simulink model "WM390_IMA_1DModel23_v2_GroupXX"  (R2021b)
settings: Solver=ode14x  StartTime=0.0  StopTime=1800  FixedStep=0.01  RelTol=1e-3
PreLoadFcn:
  | load('ACS_1DModel23_Parameters_v2.mat');
values from neighbouring files (symbols this model uses):
  AmbTemp = 25    [ACS_1DModel23_Parameters_v2.mat]
  CellContCur = 8.3    [ACS_1DModel23_Parameters_v2.mat]
  Init_SoC = 100    [ACS_1DModel23_Parameters_v2.mat]
  kI = 0.001    [ACS_1DModel23_Parameters_v2.mat]
  kP = 0.05    [ACS_1DModel23_Parameters_v2.mat]
  nP = 3    [ACS_1DModel23_Parameters_v2.mat]
  nS = 96    [ACS_1DModel23_Parameters_v2.mat]
  SoCmin = 10    [ACS_1DModel23_Parameters_v2.mat]
  ThrottleBP = [0 5 10 15 20 25 30 35 40 45 50 55 ... (21 elements, 21x1)]    [ACS_1DModel23_Parameters_v2.mat]
  TMaxMotor = 120    [ACS_1DModel23_Parameters_v2.mat]
undefined symbols (not defined in the file or in its folder): G_A, VehicleMass
libraries: nesl_utility x21, fl_lib x14, sdl_lib x8, simulink x3, autolibrcnetworksystem x1, autolibmappedmotorcommon x1, autolibshared x1
(part 1 of 2)
settings Model: PauseTimes=2  NumberOfSteps=200000  Creator=ogden.michael  LastModifiedBy=Truong Bui
settings SolverCC: AlgebraicLoopSolver=TrustRegion
settings DataIOCC: ReturnWorkspaceOutputs=off
settings OptimizationCC: EnhancedBackFolding=on  PassReuseOutputArgsThreshold=0  OptimizeBlockOrder=speed  DifferentSizesBufferReuse=on  OptimizationCustomize=off
settings DebuggingCC: AlgebraicLoopMsg=none  ParameterTunabilityLossMsg=error  SFMachineParentedDataDiag=warning  ArithmeticOperatorsInVariantConditions=warning
settings SFSimCC: SimUseLocalCustomCode=off  MATLABDynamicMemAlloc=off  CustomCodeUndefinedFunction=UseInterfaceOnly
settings RTWCC: RTWVerbose=off  RTWUseLocalCustomCode=off
settings CodeAppCC: ForceParamTrailComments=on  OperatorAnnotations=on
settings GRTTargetCC: TargetLangStandard=C89/C90 (ANSI)
settings SimscapeCC: SimscapeNormalizeSystem=off

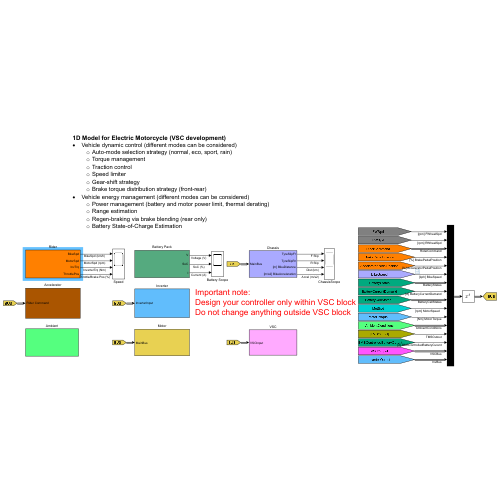
[thumbnail: Simulink's stored preview of the top-level diagram]
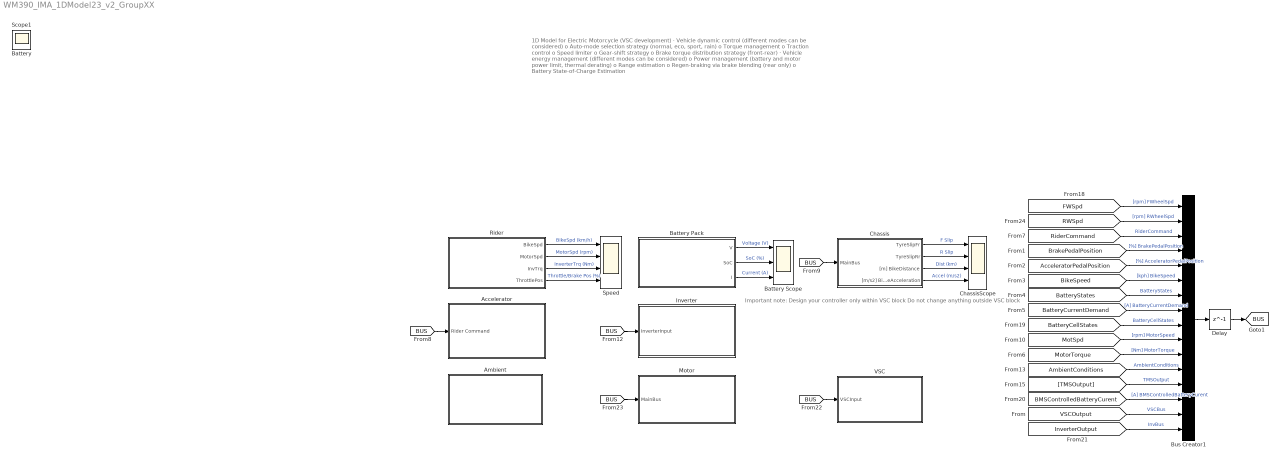
== system WM390_IMA_1DModel23_v2_GroupXX ==
  note: Important note:
      | Design your controller only within VSC block
      | Do not change anything outside VSC block
  note: 1D Model for Electric Motorcycle (VSC development)
      | · Vehicle dynamic control (different modes can be considered)
      | o Auto-mode selection strategy (normal, eco, sport, rain)
      | o Torque management
      | o Traction control
      | o Speed limiter
      | o Gear-shift strategy
      | o Brake torque distribution strategy (front-rear)
      | · Vehicle energy management (different modes can be considered)
      | o Power management (battery and motor power limit, thermal derating)
      | o Range estimation
      | o Regen-braking via brake blending (rear only)
      | o Battery State-of-Charge Estimation
  Accelerator : Subsystem
  Ambient : Subsystem
  Battery Pack : Subsystem
  Battery Scope : Scope  NumInputPorts=3
  Bus Creator1 : BusCreator  Inputs=16  OutDataTypeStr=Bus: ModelBus
      settings: InheritFromInputs=off
  Chassis : Subsystem
  ChassisScope : Scope  NumInputPorts=4
  Delay : Delay  DelayLength=1
  Inverter : Subsystem
  Motor : Subsystem
  Rider : Subsystem
  Speed : Scope  NumInputPorts=4
  VSC : Subsystem
  Battery : Scope
  Scope1 : Scope
  tag scope: BUS=global
  wires:
  [BrakePedalPosition] -> Bus Creator1/4  "[%] BrakePedalPosition"
  [AcceleratorPedalPosition] -> Bus Creator1/5  "[%] AcceleratorPedalPosition"
  [BikeSpeed] -> Bus Creator1/6  "[kph] BikeSpeed"
  [BatteryStates] -> Bus Creator1/7  "BatteryStates"
  [BatteryCurrentDemand] -> Bus Creator1/8  "[A] BatteryCurrentDemand"
  [MotorTorque] -> Bus Creator1/11  "[Nm] MotorTorque"
  [RiderCommand] -> Bus Creator1/3  "RiderCommand"
  [AmbientConditions] -> Bus Creator1/12  "AmbientConditions"
  [TMSOutput] -> Bus Creator1/13  "TMSOutput"
  [BatteryCellStates] -> Bus Creator1/9  "BatteryCellStates"
  [BMSControlledBatteryCurent] -> Bus Creator1/14  "[A] BMSControlledBatteryCurent"
  [BUS] -> Accelerator/1(Rider Command)
  [BUS] -> Inverter/1(InverterInput)
  Bus Creator1/1 -> Delay/1
  [VSCOutput] -> Bus Creator1/15  "VSCBus"
  [InverterOutput] -> Bus Creator1/16  "InvBus"
  [RWSpd] -> Bus Creator1/2  "[rpm] RWheelSpd"
  [BUS] -> Motor/1(MainBus)
  [BUS] -> VSC/1(VSCInput)
  [MotSpd] -> Bus Creator1/10  "[rpm] MotorSpeed"
  [FWSpd] -> Bus Creator1/1  "[rpm] FWheelSpd"
  Delay/1 -> [BUS]
  Chassis/3("[m] BikeDistance") -> ChassisScope/3  "Dist (km)"
  [BUS] -> Chassis/1(MainBus)
  Chassis/1(TyreSlipFr) -> ChassisScope/1  "F Slip"
  Chassis/2(TyreSlipRr) -> ChassisScope/2  "R Slip"
  Chassis/4("[m/s2] BikeAcceleration") -> ChassisScope/4  "Accel (m/s2)"
  Battery Pack/3(I) -> Battery Scope/3  "Current (A)"
  Battery Pack/2(SoC) -> Battery Scope/2  "SoC (%)"
  Battery Pack/1(V) -> Battery Scope/1  "Voltage (V)"
  Rider/3(InvTrq) -> Speed/3  "InverterTrq (Nm)"
  Rider/2(MotorSpd) -> Speed/2  "MotorSpd (rpm)"
  Rider/1(BikeSpd) -> Speed/1  "BikeSpd (km/h)"
  Rider/4(ThrottlePos) -> Speed/4  "Throttle/Brake Pos (%)"

== system WM390_IMA_1DModel23_v2_GroupXX/Accelerator ==
  Rider Command : Inport
  Accelerator Dynamics : TransferFcn  Denominator=[0.15 1]
  Accelerator Limitter : Saturate  UpperLimit=100  LowerLimit=0  ZeroCross=off
  Bus Selector : BusSelector  OutputSignals=RiderCmd.AccCmd
  tag scope: AccelCmd=global, AcceleratorPedalPosition=global
  wires:
  Accelerator Limitter/1 -> [AccelCmd], Accelerator Dynamics/1  "AcceleratorPedalPosition[%]"
  Bus Selector/1 -> Accelerator Limitter/1  "<AccCmd>"
  Rider Command/1 -> Bus Selector/1  "RiderCommand"
  Accelerator Dynamics/1 -> [AcceleratorPedalPosition]

== system WM390_IMA_1DModel23_v2_GroupXX/Ambient ==
  Ambient Temperature [C] : Constant  Value=AmbTemp
  Bus Creator : BusCreator  Inputs=2  OutDataTypeStr=Bus: AmbCondBus
      settings: InheritFromInputs=off
  Radio Button3 : RadioButtonGroup  LabelPosition=Hide  SelectedLabel=Dry  ButtonGroupName=Road Cond
      settings: Values={{'Dry', 'Wet', 'Snow', 'Ice'}, [1 2 3 4]}
  Road Condition : Constant
  tag scope: AmbientConditions=global, RoadCond=global
  wires:
  Ambient Temperature [C]/1 -> Bus Creator/1
  [RoadCond] -> Bus Creator/2
  Bus Creator/1 -> [AmbientConditions]
  Road Condition/1 -> [RoadCond]

== system WM390_IMA_1DModel23_v2_GroupXX/Battery Pack ==
  Bus Creator : BusCreator  Inputs=3  OutDataTypeStr=Bus: BattStateBus
      settings: InheritFromInputs=off
  Bus Selector1 : BusSelector  OutputSignals=AmbCond.AmbientTemps,BMSCtrlBattCurr
  Bus Selector2 : BusSelector  OutputSignals=CellVolt,CellSOC,CellTemp
  IntialSoC : Constant  Value=Init_SoC
  Single Cell Model : Subsystem
  batt2cellCurrent : Gain  Gain=1/nP
  cell2batVolt : Gain  Gain=nS
  V : Outport
  SoC : Outport  Port=2
  I : Outport  Port=3
  tag scope: BatteryStates=global
  wires:
  IntialSoC/1 -> Single Cell Model/3(Initial SoC)
  batt2cellCurrent/1 -> I/1, Single Cell Model/2(BatteryCellCurrent)
  cell2batVolt/1 -> Bus Creator/1  "BattVolt"
  Bus Selector1/2 -> batt2cellCurrent/1  "<BMSCtrlBattCurr>"
  Bus Selector2/1 -> V/1, cell2batVolt/1  "<CellVolt>"
  Bus Selector1/1 -> Single Cell Model/1(Temp)  "<AmbientTemps>"
  Single Cell Model/1(Cell State) -> Bus Selector2/1
  [BUS] -> Bus Selector1/1
  Bus Selector2/2 -> SoC/1, Bus Creator/2  "<CellSOC>"
  Bus Creator/1 -> [BatteryStates]
  Bus Selector2/3 -> Bus Creator/3  "<CellTemp>"

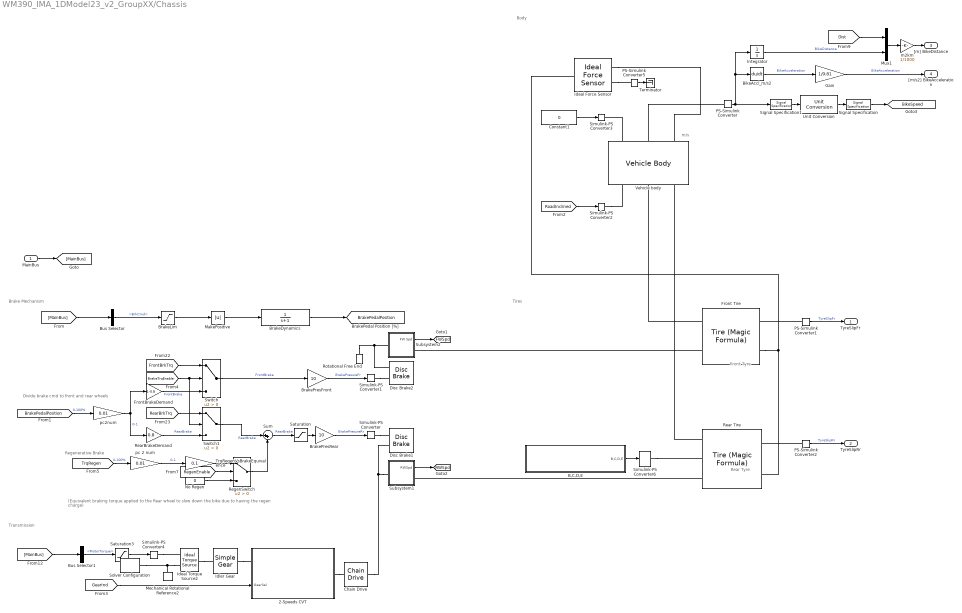
== system WM390_IMA_1DModel23_v2_GroupXX/Chassis ==
  note: Regenerative Brake
  note: Transmission
  note: Body
  note: Tires
  note: Brake Mechanism
  note: Divide brake cmd to front and rear wheels
  note: Rear Tyre
  note: Front Tyre
  note: m/s
  note: (Equivalent braking torque applied to the Rear wheel to slow down the bike due to having the regen charge)
  MainBus : Inport
  2-Speeds CVT : Subsystem
      settings: PortSchema="{\"entries\":[{\"content\":{\"sides\":[{\"content\":{\"connectorIds\":[\"LConn1\",\"In1\"]},\"type\":\"ConnectorPlacement.EquallySpacedRectSide\",\"uuid\":\"b79ba6b3-25f2-43ad-8d13-28516f3c2dbb\"},{\"content\":{\"connectorIds\":[\"RConn1\"],\"side\":\"RIGHT\"},\"type\":\"ConnectorPlacement.EquallySpacedRectSide\",\"uuid\":\"f2f7b57b-224a-4cc2-9c38-49f8210c3cf7\"},{\"content\":{\"connectorIds\":[],\"side\":\"TOP\"},\"type\":\"ConnectorPlacement.EquallySpacedRectSide\",\"uuid\":\"abb9111b-7a6e-41b3-84ac-3885d12f9cc0\"}]},\"type\":\"ConnectorPlacement.EquallySpacedConnector\",\"uuid\":\"ff58775e-0d64-43a4-a5c7-d5e7a3ebae26\"}],\"packageUris\":[\"http://schema.mathworks.com/mf0/Connector/R2020b\"],\"version\":\"1.0\"}"
  B,C,D,E : Subsystem
  BikeAccl_m/s2 : Derivative
  BrakeDynamics : TransferFcn  Denominator=[1 1]
  BrakeLim : Saturate  UpperLimit=0  LowerLimit=-100
  BrakePresFront : Gain  Gain=10
  BrakePresRear : Gain  Gain=10
  Bus Selector : BusSelector  OutputSignals=RiderCmd.BrkCmd
  Bus Selector1 : BusSelector  OutputSignals=MotorTorque
  Chain Drive : sdl_lib/Couplings & Drives/Chain Drive  chain_model=sdl.enum.chain_model.ideal  radius_a=15 mm  radius_b=45 mm  slack=50 mm  k_chain=1e5 N/m  mu_visc_chain=5 N/(m/s)  mu_visc_a=0.001 N*m/(rad/s)  mu_visc_b=0.001 N*m/(rad/s)  breakable=sdl.enum.max_tension.off  F_max=1e6 N  x_specify=off  x_priority=High  x=0 mm  x_nominal_specify=off  x_nominal_unit=mm  x_nominal_value=1
      settings: SourceProductBaseCode=LD  InternalSimscapePortConfiguration="{\"Bottom\":[],\"Left\":[{\"id\":\"A\",\"label\":\"A\",\"type\":\"foundation.mechanical.rotational.rotational\"}],\"Right\":[{\"id\":\"B\",\"label\":\"B\",\"type\":\"foundation.mechanical.rotational.rotational\"}],\"Top\":[]}"
  Constant1 : Constant  Value=0
  Disc Brake1 : sdl_lib/Brakes & Detents/Rotational/Disc Brake  r_mean=170 mm  bore=60 mm  n_pads=2  thermal_port=simscape.enum.thermaleffects.omit  mu_static=0.9  mu_coulomb=0.7  temperature_TLU=[280, 300, 320] K  mu_static_TLU=[.9, .8, .7]  mu_coulomb_TLU=[.8, .7, .6]  brkwy_vel=0.1 rad/s  visc_coef=.001 N*m/(rad/s)  enable_faults=simscape.enum.onoff.off  faulted_pressure=0 bar  external_fault=simscape.enum.onoff.off  temporal_fault=simscape.enum.onoff.off  fault_time=5 s  report_fault=simscape.enum.assert.action.none  thermal_mass=50 kJ/K  temperature_specify=off  temperature_priority=High  temperature=300 K  temperature_nominal_specify=off  temperature_nominal_unit=K  temperature_nominal_value=1
      settings: SourceProductBaseCode=LD
  Disc Brake2 : sdl_lib/Brakes & Detents/Rotational/Disc Brake  r_mean=170 mm  bore=60 mm  n_pads=2  thermal_port=simscape.enum.thermaleffects.omit  mu_static=0.9  mu_coulomb=0.7  temperature_TLU=[280, 300, 320] K  mu_static_TLU=[.9, .8, .7]  mu_coulomb_TLU=[.8, .7, .6]  brkwy_vel=0.1 rad/s  visc_coef=.001 N*m/(rad/s)  enable_faults=simscape.enum.onoff.off  faulted_pressure=0 bar  external_fault=simscape.enum.onoff.off  temporal_fault=simscape.enum.onoff.off  fault_time=5 s  report_fault=simscape.enum.assert.action.none  thermal_mass=50 kJ/K  temperature_specify=off  temperature_priority=High  temperature=300 K  temperature_nominal_specify=off  temperature_nominal_unit=K  temperature_nominal_value=1
      settings: SourceProductBaseCode=LD
  Front Tire : sdl_lib/Tires & Vehicles/Tire (Magic Formula)  parameterization=sdl.enum.magic_tire_model.peak  F_z1=2000 N  F_x1=5000 N  kappa1=10  B_m=10  C_m=1.9  D_m=1  E_m=0.97  fz0=4000 N  p_Cx=1.685  p_Dx=[1.21, -.037]  p_Ex=[.344, .095, -.02, 0]  p_Kx=[21.51, -.163, .245]  p_Hx=[-.002, .002]  p_Vx=[0, 0]  r_e=0.32 m  model_compliance=sdl.enum.compliance.off  stiffness=1e6 N/m  damping=1000 N/(m/s)  model_inertia=sdl.enum.model_inertia.off  inertia=0.2 kg*m^2  initial_velocity=0 rad/s  model_resistance=simscape.enum.onoff.off  resistance_model=sdl.enum.rollingResistanceParameterization.constant  coeff=0.015  p_tire=250e3 Pa  alpha=-0.003  beta=0.97  coeff_a=84e-4  coeff_b=6.2e-4 s/m  coeff_c=1.6e-4 s^2/m^2  v_thr=0.001 m/s  v_tr_thr=0.1 m/s
  FrontBrakeDemand : Gain  Gain=1-0.8
  Gain : Gain  Gain=1/9.81
  Ideal Force Sensor : fl_lib/Mechanical/Mechanical Sensors/Ideal Force Sensor
  Ideal Torque Source2 : fl_lib/Mechanical/Mechanical Sources/Ideal Torque Source
  Idler Gear : sdl_lib/Gears/Simple Gear  ratio=1  rotation_direction=sdl.enum.shaftOutputDirection.opposite  friction_model=sdl.enum.gear_efficiencies_load.constant  T_noload=0.1 N*m  T_nom=5 N*m  efficiency_nom=0.8  efficiency=0.8845  temperature_TLU=[280, 300, 320] K  load_TLU=[1, 5, 10] N*m  efficiency_TLU=[.95, .9, .85]  efficiency_TLU2=[.85, .8, .75; .95, .9, .85; .85, .8, .7]  w_thr=0.01 rad/s  pwr_thr=0.001 W  backlash_model=sdl.enum.backlashModel.Off  backlash_distance=1e-3 mm  x0=0 mm  r_base=0.1 m  hardstop_model=simscape.enum.hardstop.smooth  transition=1e-4 mm  backlash_stiffness=1e7 N/m  backlash_damping=1e6 N/(m/s)  e=0  v_tol=0.001 m/s  mu_visc=[0, 0] N*m/(rad/s)  enable_faults=simscape.enum.onoff.off  efficiency_fault=0.05  external_fault=simscape.enum.onoff.off  temporal_fault=simscape.enum.onoff.off  fault_time=5 s  fault_angles=pi / 12 rad  report_fault=simscape.enum.assert.action.none  thermal_mass=50 J/K  temperature_specify=off  temperature_priority=High  temperature=300 K  temperature_nominal_specify=off  temperature_nominal_unit=K  temperature_nominal_value=1  x_backlash_specify=off  x_backlash_priority=None  x_backlash=0 mm  x_backlash_nominal_specify=off  x_backlash_nominal_unit=mm  x_backlash_nominal_value=1  f_hardstop_specify=off  f_hardstop_priority=None  f_hardstop=0 N  f_hardstop_nominal_specify=off  f_hardstop_nominal_unit=N  f_hardstop_nominal_value=1  v_backlash_specify=off  v_backlash_priority=None  v_backlash=0 m/s  v_backlash_nominal_specify=off  v_backlash_nominal_unit=m/s  v_backlash_nominal_value=1
  Integrator : Integrator
  MakePositive : Abs
  Mechanical Rotational Reference2 : fl_lib/Mechanical/Rotational Elements/Mechanical Rotational Reference
  Mux1 : Mux  Inputs=2
  No Regen : Constant  Value=0
  PS-Simulink Converter : nesl_utility/PS-Simulink Converter  PhysicalDomain=network_engine_domain  SubClassName=ps_output  LeftPortType=input  RightPortType=output  PseudoPeriodic=off  Frequencies=[]  Unit=m/s  AffineConversion=off
      settings: SourceProductBaseCode=PW,SS
  PS-Simulink Converter1 : nesl_utility/PS-Simulink Converter  PhysicalDomain=network_engine_domain  SubClassName=ps_output  LeftPortType=input  RightPortType=output  PseudoPeriodic=off  Frequencies=[]  Unit=rpm  AffineConversion=off
      settings: SourceProductBaseCode=PW,SS
  PS-Simulink Converter2 : nesl_utility/PS-Simulink Converter  PhysicalDomain=network_engine_domain  SubClassName=ps_output  LeftPortType=input  RightPortType=output  PseudoPeriodic=off  Frequencies=[]  Unit=rpm  AffineConversion=off
      settings: SourceProductBaseCode=PW,SS
  PS-Simulink Converter5 : nesl_utility/PS-Simulink Converter  PhysicalDomain=network_engine_domain  SubClassName=ps_output  LeftPortType=input  RightPortType=output  PseudoPeriodic=off  Frequencies=[]  Unit=inherit  AffineConversion=off
      settings: SourceProductBaseCode=PW,SS
  Rear Tire : sdl_lib/Tires & Vehicles/Tire (Magic Formula)  parameterization=sdl.enum.magic_tire_model.PS  F_z1=R_V_Load N  F_x1=Peak_LForce_R N  kappa1=Slp_prc  B_m=10  C_m=1.9  D_m=1  E_m=0.97  fz0=4000 N  p_Cx=1.685  p_Dx=[1.21, -.037]  p_Ex=[.344, .095, -.02, 0]  p_Kx=[21.51, -.163, .245]  p_Hx=[-.002, .002]  p_Vx=[0, 0]  r_e=0.32 m  model_compliance=sdl.enum.compliance.off  stiffness=1e6 N/m  damping=1000 N/(m/s)  model_inertia=sdl.enum.model_inertia.off  inertia=0.2 kg*m^2  initial_velocity=0 rad/s  model_resistance=simscape.enum.onoff.on  resistance_model=sdl.enum.rollingResistanceParameterization.constant  coeff=0.015  p_tire=250e3 Pa  alpha=-0.003  beta=0.97  coeff_a=84e-4  coeff_b=6.2e-4 s/m  coeff_c=1.6e-4 s^2/m^2  v_thr=0.001 m/s  v_tr_thr=0.1 m/s
      settings: InternalSimscapePortConfiguration="{\"Bottom\":[],\"Left\":[{\"id\":\"N\",\"label\":\"N\",\"type\":\"input\"},{\"id\":\"M\",\"label\":\"M\",\"type\":\"input\"},{\"id\":\"A\",\"label\":\"A\",\"type\":\"foundation.mechanical.rotational.rotational\"}],\"Right\":[{\"id\":\"S\",\"label\":\"S\",\"type\":\"output\"},{\"id\":\"H\",\"label\":\"H\",\"type\":\"foundation.mechanical.translational.translational\"}],\"Top\":[]}"
  RearBrakeDemand : Gain  Gain=0.8
  RegenSwitch : Switch  Criteria=u2 > Threshold
  Rotational Free End : fl_lib/Mechanical/Rotational Elements/Rotational Free End  w_specify=off  w_priority=None  w=0 rad/s  w_nominal_specify=off  w_nominal_unit=rad/s  w_nominal_value=1
      settings: SourceProductBaseCode=SS
  Saturation : Saturate  UpperLimit=1  LowerLimit=0
  Saturation3 : Saturate  UpperLimit=TMaxMotor  LowerLimit=-15
  Signal Specification : SignalSpecification  Unit=km/hr
  Signal Specification1 : SignalSpecification  Unit=m/s
  Simulink-PS Converter : nesl_utility/Simulink-PS Converter  PhysicalDomain=network_engine_domain  SubClassName=ps_input  LeftPortType=input  RightPortType=output  PseudoPeriodic=off  Frequencies=[]  NoiseDistribution=none  NoiseParameters=[]  Unit=bar  AffineConversion=off  FilteringAndDerivatives=filter  SimscapeFilterOrder=1  InputFilterTimeConstant=0.001  UdotUserProvided=0
      settings: SourceProductBaseCode=PW,SS
  Simulink-PS Converter1 : nesl_utility/Simulink-PS Converter  PhysicalDomain=network_engine_domain  SubClassName=ps_input  LeftPortType=input  RightPortType=output  PseudoPeriodic=off  Frequencies=[]  NoiseDistribution=none  NoiseParameters=[]  Unit=bar  AffineConversion=off  FilteringAndDerivatives=filter  SimscapeFilterOrder=1  InputFilterTimeConstant=0.001  UdotUserProvided=0
      settings: SourceProductBaseCode=PW,SS
  Simulink-PS Converter2 : nesl_utility/Simulink-PS Converter  PhysicalDomain=network_engine_domain  SubClassName=ps_input  LeftPortType=input  RightPortType=output  PseudoPeriodic=off  Frequencies=[]  NoiseDistribution=none  NoiseParameters=[]  Unit=1  AffineConversion=off  FilteringAndDerivatives=provide  SimscapeFilterOrder=1  InputFilterTimeConstant=0.001  UdotUserProvided=0
      settings: SourceProductBaseCode=PW,SS
  Simulink-PS Converter3 : nesl_utility/Simulink-PS Converter  PhysicalDomain=network_engine_domain  SubClassName=ps_input  LeftPortType=input  RightPortType=output  PseudoPeriodic=off  Frequencies=[]  NoiseDistribution=none  NoiseParameters=[]  Unit=1  AffineConversion=off  FilteringAndDerivatives=provide  SimscapeFilterOrder=1  InputFilterTimeConstant=0.001  UdotUserProvided=0
      settings: SourceProductBaseCode=PW,SS
  Simulink-PS Converter4 : nesl_utility/Simulink-PS Converter  PhysicalDomain=network_engine_domain  SubClassName=ps_input  LeftPortType=input  RightPortType=output  PseudoPeriodic=off  Frequencies=[]  NoiseDistribution=none  NoiseParameters=[]  Unit=1  AffineConversion=off  FilteringAndDerivatives=provide  SimscapeFilterOrder=1  InputFilterTimeConstant=0.001  UdotUserProvided=0
      settings: SourceProductBaseCode=PW,SS
  Simulink-PS Converter6 : nesl_utility/Simulink-PS Converter  PhysicalDomain=network_engine_domain  SubClassName=ps_input  LeftPortType=input  RightPortType=output  PseudoPeriodic=off  Frequencies=[]  NoiseDistribution=none  NoiseParameters=[]  Unit=1  AffineConversion=off  FilteringAndDerivatives=filter  SimscapeFilterOrder=1  InputFilterTimeConstant=0.05  UdotUserProvided=0
      settings: SourceProductBaseCode=PW,SS
  Solver Configuration : nesl_utility/Solver Configuration  PhysicalDomain=network_engine_domain  SubClassName=solver  LeftPortType=input  RightPortType=generic  Tones=[]  Harmonics=[]  SimulateNoise=off  Profile=off  UseLocalSampling=off  EnableSwitchedLinearOptims=on  FrequencyDomain=off  UseCCode=off  RelTol=0.001  AbsTol=1e-06  MinStep=1e-09  ToWorkspace=off  RevertToSquareIcSolve=off  NumHomotopyIterations=100  PhasorMode=off  PhasorModeNumHarmonics=1  DoDC=off  ResidualTolerance=1e-9  UseLocalSolver=on  LocalSolverChoice=NE_BACKWARD_EULER_ADVANCER  LocalSolverSampleTime=0.01  DoFixedCost=on  MaxNonlinIter=3  MaxModeIter=2  ComputeImpulses=off  ImpulseIterations=2  LinearAlgebra=Full  EquationFormulation=NE_TIME_EF  DelaysMemoryBudget=1024  AutomaticFiltering=on  FilteringTimeConstant=0.001  PartitionStorageMethod=AS_NEEDED  PartitionMemoryBudget=1024  PartitionMethod=ROBUST
      settings: SourceProductBaseCode=PW,SS
  Subsystem1 : Subsystem
      mask Display: disp('Rotational\nSensor 4')
  Subsystem2 : Subsystem
      mask Display: disp('Rotational\nSensor 5')
  Sum : Sum  Inputs=|++
  Switch : Switch  Criteria=u2 > Threshold
  Switch1 : Switch  Criteria=u2 > Threshold
  Terminator : Terminator
  TrqRegenVsBrakeEquivalence : Gain  Gain=0.1
  Unit Conversion : UnitConversion
  Vehicle body : sdl_lib/Tires & Vehicles/Vehicle Body  mass=250+80 kg  n_w=1  x_f=0.7 m  x_r=0.7 m  y_c=0.585 m  mass_var=simscape.enum.onoff.off  g=9.81 m/s^2  liftoff_warning=simscape.enum.onoff.off  area=0.74 m^2  Cd=0.7  rho=1.225 kg/m^3  model_pitch=simscape.enum.onoff.on  inertia=4000 kg*m^2  suspension_model=sdl.enum.linearTLU.linear  k_f=10000 N/m  b_f=10000 N/(m/s)  k_r=10000 N/m  b_r=10000 N/(m/s)  k_f_TLU=[-2000, -1000, 0, 1000, 2000] N  x_f_TLU=[-.4, -.2, 0, .2, .4] m  b_f_TLU=[-200, -100, 0, 100, 200] N  v_f_TLU=[-4, -2, 0, 2, 4] m/s  k_r_TLU=[-2000, -1000, 0, 1000, 2000] N  x_r_TLU=[-.4, -.2, 0, .2, .4] m  b_r_TLU=[-200, -100, 0, 100, 200] N  v_r_TLU=[-4, -2, 0, 2, 4] m/s  interp_method=simscape.enum.interpolation.linear  extrap_method=simscape.enum.extrapolation.linear  model_hardstop=simscape.enum.onoff.off  upper_bound_f=.25 m  lower_bound_f=-.25 m  stop_k_f=1e6 N/m  stop_b_f=150 N/(m/s)  upper_bound_r=.25 m  lower_bound_r=-.25 m  stop_k_r=1e6 N/m  stop_b_r=150 N/(m/s)  initial_pitch=0 rad  initial_pitch_rate=0 rad/s  v_specify=off  v_priority=High  v=0 m/s  v_nominal_specify=off  v_nominal_unit=m/s  v_nominal_value=1
  m2km : Gain  Gain=1/1000
  pc 2 num : Gain  Gain=0.01
  pc2num : Gain  Gain=0.01
  TyreSlipFr : Outport
  TyreSlipRr : Outport  Port=2
  "[m] BikeDistance" : Outport  Port=3
  "[m/s2] BikeAcceleration" : Outport  Port=4
  tag scope: BikeSpeed=global, BrakePedalPosition=global, FWSpd=global, RWSpd=global
  wires:
  Sum/1 -> Saturation/1  "RearBrake"
  Switch/1 -> BrakePresFront/1  "FrontBrake"
  [BrakePedalPosition] -> pc2num/1  "0-100%"
  pc2num/1 -> RearBrakeDemand/1, FrontBrakeDemand/1  "0-1"
  MakePositive/1 -> BrakeDynamics/1
  BrakePresRear/1 -> Simulink-PS Converter/1  "BrakePresureRr"
  BrakeLim/1 -> MakePositive/1
  BrakeDynamics/1 -> [BrakePedalPosition]
  Bus Selector/1 -> BrakeLim/1  "<BrkCmd>"
  BrakePresFront/1 -> Simulink-PS Converter1/1  "BrakePresureFr"
  MainBus/1 -> [MainBus]
  [MainBus] -> Bus Selector/1
  PS-Simulink Converter1/1 -> TyreSlipFr/1  "TyreSlipFr"
  B,C,D,E/1(B,C,D,E) -> Simulink-PS Converter6/1
  PS-Simulink Converter2/1 -> TyreSlipRr/1  "TyreSlipRr"
  Constant1/1 -> Simulink-PS Converter3/1
  Integrator/1 -> Mux1/2  "BikeDistance"
  BikeAccl_m/s2/1 -> Gain/1  "BikeAcceleration"
  Gain/1 -> "[m/s2] BikeAcceleration"/1  "BikeAcceleration"
  PS-Simulink Converter5/1 -> Terminator/1
  Mux1/1 -> m2km/1
  PS-Simulink Converter/1 -> BikeAccl_m/s2/1, Integrator/1, Signal Specification1/1
  Signal Specification1/1 -> Unit Conversion/1
  [RoadInclined] -> Simulink-PS Converter2/1
  Signal Specification/1 -> [BikeSpeed]
  [Dist] -> Mux1/1
  Unit Conversion/1 -> Signal Specification/1
  Bus Selector1/1 -> Saturation3/1  "<MotorTorque>"
  [MainBus] -> Bus Selector1/1
  [GearInd] -> 2-Speeds CVT/1(GearSel)
  Switch1/1 -> Sum/1  "RearBrake"
  pc 2 num/1 -> TrqRegenVsBrakeEquivalence/1  "0-1"
  [TrqRegen] -> pc 2 num/1  "0-100%"
  TrqRegenVsBrakeEquivalence/1 -> RegenSwitch/1
  Saturation/1 -> BrakePresRear/1
  FrontBrakeDemand/1 -> Switch/3  "FrontBrake"
  RearBrakeDemand/1 -> Switch1/3  "RearBrake"
  [RearBrkTrq] -> Switch1/1
  [FrontBrkTrq] -> Switch/1
  [BrakeTrqEnable] -> Switch1/2, Switch/2
  Subsystem1/1(RWSpd) -> [RWSpd]
  Subsystem2/1(FW Spd) -> [FWSpd]
  Saturation3/1 -> Simulink-PS Converter4/1
  m2km/1 -> "[m] BikeDistance"/1
  [RegenEnable] -> RegenSwitch/2
  No Regen/1 -> RegenSwitch/3
  RegenSwitch/1 -> Sum/2
  connections:
  Rotational Free End/LConn1 -- Subsystem2/LConn1 -- Disc Brake2/LConn2
  Subsystem1/LConn1 -- Chain Drive/RConn1 -- Disc Brake1/LConn2
  Front Tire/LConn2 -- Subsystem2/RConn1
  Simulink-PS Converter1/RConn1 -- Disc Brake2/LConn1
  Simulink-PS Converter/RConn1 -- Disc Brake1/LConn1
  Rear Tire/LConn3 -- Subsystem1/RConn1
  PS-Simulink Converter2/LConn1 -- Rear Tire/RConn1
  PS-Simulink Converter1/LConn1 -- Front Tire/RConn1
  Simulink-PS Converter6/RConn1 -- Rear Tire/LConn2
  Front Tire/LConn1 -- Vehicle body/RConn2
  Rear Tire/LConn1 -- Vehicle body/RConn1
  Front Tire/RConn2 -- Rear Tire/RConn2 -- Ideal Force Sensor/LConn1
  Ideal Force Sensor/RConn2 -- PS-Simulink Converter5/LConn1
  Vehicle body/LConn2 -- PS-Simulink Converter/LConn1
  Vehicle body/LConn3 -- Simulink-PS Converter3/RConn1
  Ideal Force Sensor/RConn1 -- Vehicle body/LConn1
  Simulink-PS Converter2/RConn1 -- Vehicle body/RConn3
  Ideal Torque Source2/RConn2 -- Mechanical Rotational Reference2/LConn1 -- Solver Configuration/RConn1
  Ideal Torque Source2/LConn1 -- Idler Gear/LConn1
  Idler Gear/RConn1 -- 2-Speeds CVT/LConn1
  2-Speeds CVT/RConn1 -- Chain Drive/LConn1
  Simulink-PS Converter4/RConn1 -- Ideal Torque Source2/RConn1

== system WM390_IMA_1DModel23_v2_GroupXX/Inverter ==
  InverterInput : Inport
  Bus Creator : BusCreator  Inputs=3  OutDataTypeStr=Bus: INVBus
  Bus Selector : BusSelector  OutputSignals=VSCBus.TrqFCmd,RWheelSpd,MotorTorque
  Efficiency and Powerloss Calculation : Subsystem
  Inv Transfer Func : Gain
  Product1 : Product
  RegenSwitch : Switch  Criteria=u2 > Threshold
  Transmission : Subsystem
  tag scope: InverterOutput=global
  wires:
  InverterInput/1 -> Bus Selector/1
  Efficiency and Powerloss Calculation/2(PwrLoss) -> Bus Creator/3  "invP_loss_W"
  Bus Selector/3 -> Efficiency and Powerloss Calculation/2(Trq)  "<MotorTorque>"
  Bus Creator/1 -> [InverterOutput]
  Bus Selector/1 -> RegenSwitch/3  "<TrqFCmd>"
  Efficiency and Powerloss Calculation/1(eff) -> Bus Creator/2
  Inv Transfer Func/1 -> Bus Creator/1
  Bus Selector/2 -> Product1/1  "<RWheelSpd>"
  Transmission/1(Transmission) -> Product1/2
  RegenSwitch/1 -> Inv Transfer Func/1
  [TrqRegen] -> RegenSwitch/1
  [RegenEnable] -> RegenSwitch/2
  Product1/1 -> Efficiency and Powerloss Calculation/1(Spd)

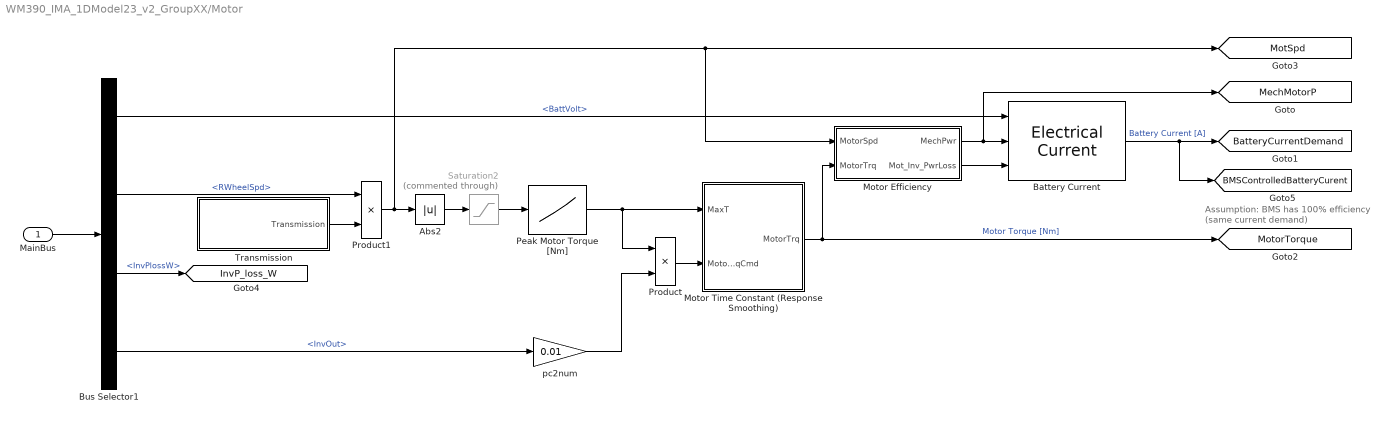
== system WM390_IMA_1DModel23_v2_GroupXX/Motor ==
  note: Assumption: BMS has 100% efficiency
      | (same current demand)
  MainBus : Inport
  Abs2 : Abs
  Battery Current : autolibmappedmotorcommon/Electrical Current  SystemSampleTime=-1  VariantActivationTime=update diagram  Latency=0  AutoFrameSizeCalculation=off
      settings: SourceProductBaseCode=PW,DR,MT,UV,VE
  Bus Selector1 : BusSelector  OutputSignals=BatteryStates.BattVolt,RWheelSpd,InvBus.InvPlossW,InvBus.InvOut
  Motor Efficiency : Subsystem
  Motor Time Constant (Response Smoothing) : Subsystem
  Peak Motor Torque [Nm] : Lookup_n-D  NumberOfTableDimensions=1  BreakpointsForDimension1=[0 2000 5000 7000]  Table=[120 115 95 70]  ExtrapMethod=Clip  InternalRulePriority=Speed  RndMeth=Simplest  InputSameDT=on
  Product : Product
  Product1 : Product
  Saturation2 : Saturate  Commented=through  UpperLimit=7000  LowerLimit=-7000
  Transmission : Subsystem
  pc2num : Gain  Gain=0.01
  tag scope: BMSControlledBatteryCurent=global, BatteryCurrentDemand=global, InvP_loss_W=global, MechMotorP=global, MotSpd=global, MotorTorque=global
  wires:
  Product/1 -> Motor Time Constant (Response Smoothing)/2(MotorTrqCmd)
  Bus Selector1/2 -> Product1/1  "<RWheelSpd>"
  Battery Current/1 -> [BMSControlledBatteryCurent], [BatteryCurrentDemand]  "Battery Current [A]"
  Bus Selector1/1 -> Battery Current/1  "<BattVolt>"
  MainBus/1 -> Bus Selector1/1
  Motor Efficiency/1(MechPwr) -> [MechMotorP], Battery Current/2
  Motor Time Constant (Response Smoothing)/1(MotorTrq) -> [MotorTorque], Motor Efficiency/2(MotorTrq)  "Motor Torque [Nm]"
  pc2num/1 -> Product/2
  Motor Efficiency/2(Mot_Inv_PwrLoss) -> Battery Current/3
  Transmission/1(Transmission) -> Product1/2
  Bus Selector1/3 -> [InvP_loss_W]  "<InvPlossW>"
  Bus Selector1/4 -> pc2num/1  "<InvOut>"
  Product1/1 -> Abs2/1, Motor Efficiency/1(MotorSpd), [MotSpd]
  Abs2/1 -> Saturation2/1
  Peak Motor Torque [Nm]/1 -> Product/1, Motor Time Constant (Response Smoothing)/1(MaxT)
  Saturation2/1 -> Peak Motor Torque [Nm]/1

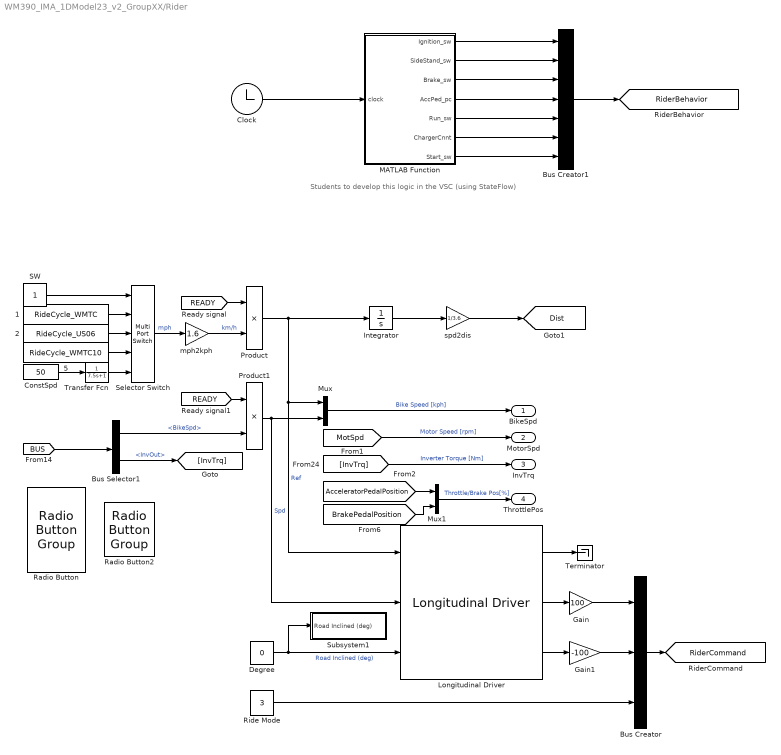
== system WM390_IMA_1DModel23_v2_GroupXX/Rider ==
  note: Students to develop this logic in the VSC (using StateFlow)
  " 1" : FromWorkspace  Tag=DriveCycle  VariableName=RideCycle_WMTC
  " 2" : FromWorkspace  Tag=DriveCycle  VariableName=RideCycle_US06
  " 5" : FromWorkspace  Tag=DriveCycle  VariableName=RideCycle_WMTC10
  Bus Creator : BusCreator  Inputs=3  OutDataTypeStr=Bus: RiderCmdBus
      settings: InheritFromInputs=off
  Bus Creator1 : BusCreator  Inputs=7  OutDataTypeStr=Bus: RiderBehBus
      settings: InheritFromInputs=off
  Bus Selector1 : BusSelector  OutputSignals=BikeSpd,InvBus.InvOut
  Clock : Clock
  ConstSpd : Constant  Value=50
  Degree : Constant  Value=0
  Gain : Gain  Gain=100
  Gain1 : Gain  Gain=-100
  Integrator : Integrator
  Longitudinal Driver : autolibshared/Longitudinal Driver  extAccelOvr=off  extDecelOvr=off  extAccelHld=off  extDecelHld=off  extAccelZero=off  extDecelZero=off  cntrlType=PI  shftType=None  velUnits=km/hr  gearOut=off  Kp=kP  Ki=kI  Kff=0  Kg=0  VehVelVec=[0 100]  KffVec=[0 0]  KpVec=[0.001 10]  KiVec=[0 0]  KgVec=[0 0]  m=VehicleMass  Kpt=0.5*VehicleMass*G_A/4  tau=0.01  L=10  aR=200  bR=1  cR=DragCoef  g=G_A  vnom=1  Kaw=0  tauerr=.03  tauPt=2  GearInit=0  tShift=.1  pdlVec=[0.1 0.4 0.5 0.9]  upShftTbl=[-1 12.9375 26.4375 39.9375 51.18749999999999 62.4375 72.84375 83.25;-1 16.3125 29.8125 43.3125 54.5624 65.8125 76.78125 87.75;-1 19.6875 33.1875 46.68749999999999 57.9375 69.1875 80.71875 92.25;-1 33 52.5 77.25 100.5 138.75 161.875 185]  dwnShftTbl=[1 9.5625 23.0625 36.5625 47.8125 59.0625 68.90625 78.75;1 12.9375 26.4375 39.9375 51.18749999999999 62.4375 72.84375 83.25;1 16.3125 29.8125 43.3125 54.562499 65.8125 76.78125 87.75;1 19.6875 33.1875 46.68749999999999 57.9375 69.1875 80.71875 92.25]  tClutch=.5  tRev=.5  tPark=120  aMode=1  UpGearVec="[0  1  2  3  4  5  6  7]"  DownGearVec="[1  2  3  4  5  6  7  8]"
      settings: SourceProductBaseCode=PW,DR,MT,UV,VE
  MATLAB Function : MATLAB Function  TreatAsAtomicUnit=on
  Mux : Mux  Inputs=2
  Mux1 : Mux  Inputs=2
  Product : Product
  Product1 : Product
  Radio Button : RadioButtonGroup  LabelPosition=Hide  SelectedLabel=Normal  ButtonGroupName=Ride Mode
      settings: Values={{'Rain', 'Eco', 'Normal', 'Sport'}, [1 2 3 4]}
  Radio Button2 : RadioButtonGroup  LabelPosition=Hide  SelectedLabel=Gear 1  ButtonGroupName=Gear Sel
      settings: Values={{'Gear 1', 'Gear 2'}, [1 2]}
  Ride Mode : Constant  Value=3
  SW : Constant
  Selector Switch : MultiPortSwitch  Inputs=4
  Subsystem1 : Subsystem
  Terminator : Terminator
  Transfer Fcn : TransferFcn  Denominator=[7.5 1]
  mph2kph : Gain  Gain=1.6
  spd2dis : Gain  Gain=1/3.6
  BikeSpd : Outport
  MotorSpd : Outport  Port=2
  InvTrq : Outport  Port=3
  ThrottlePos : Outport  Port=4
  tag scope: Dist=global, RiderBehavior=global, RiderCommand=global
  wires:
  SW/1 -> Selector Switch/1
  " 2"/1 -> Selector Switch/3
  [BUS] -> Bus Selector1/1
  Clock/1 -> MATLAB Function/1(clock)
  Degree/1 -> Subsystem1/1(Road Inclined (deg)), Longitudinal Driver/3  "Road Inclined (deg)"
  Selector Switch/1 -> mph2kph/1  "mph"
  [READY] -> Product/1
  Bus Selector1/1 -> Product1/2  "<BikeSpd>"
  [READY] -> Product1/1
  Product1/1 -> Longitudinal Driver/2, Mux/2  "Spd"
  Bus Creator/1 -> [RiderCommand]
  Longitudinal Driver/1 -> Terminator/1
  MATLAB Function/1(Ignition_sw) -> Bus Creator1/1
  MATLAB Function/2(SideStand_sw) -> Bus Creator1/2
  MATLAB Function/3(Brake_sw) -> Bus Creator1/3
  MATLAB Function/4(AccPed_pc) -> Bus Creator1/4
  MATLAB Function/5(Run_sw) -> Bus Creator1/5
  MATLAB Function/6(ChargerCnnt) -> Bus Creator1/6
  MATLAB Function/7(Start_sw) -> Bus Creator1/7
  Bus Creator1/1 -> [RiderBehavior]
  Mux/1 -> BikeSpd/1  "Bike Speed [kph]"
  Ride Mode/1 -> Bus Creator/3
  Product/1 -> Integrator/1, Longitudinal Driver/1, Mux/1  "Ref"
  Longitudinal Driver/2 -> Gain/1
  Longitudinal Driver/3 -> Gain1/1
  mph2kph/1 -> Product/2  "km/h"
  " 1"/1 -> Selector Switch/2
  " 5"/1 -> Selector Switch/4
  Integrator/1 -> spd2dis/1
  spd2dis/1 -> [Dist]
  [MotSpd] -> MotorSpd/1  "Motor Speed [rpm]"
  Mux1/1 -> ThrottlePos/1  "Throttle/Brake Pos[%]"
  [InvTrq] -> InvTrq/1  "Inverter Torque [Nm]"
  ConstSpd/1 -> Transfer Fcn/1
  Bus Selector1/2 -> [InvTrq]  "<InvOut>"
  Gain/1 -> Bus Creator/1
  Gain1/1 -> Bus Creator/2
  Transfer Fcn/1 -> Selector Switch/5
  [AcceleratorPedalPosition] -> Mux1/1
  [BrakePedalPosition] -> Mux1/2

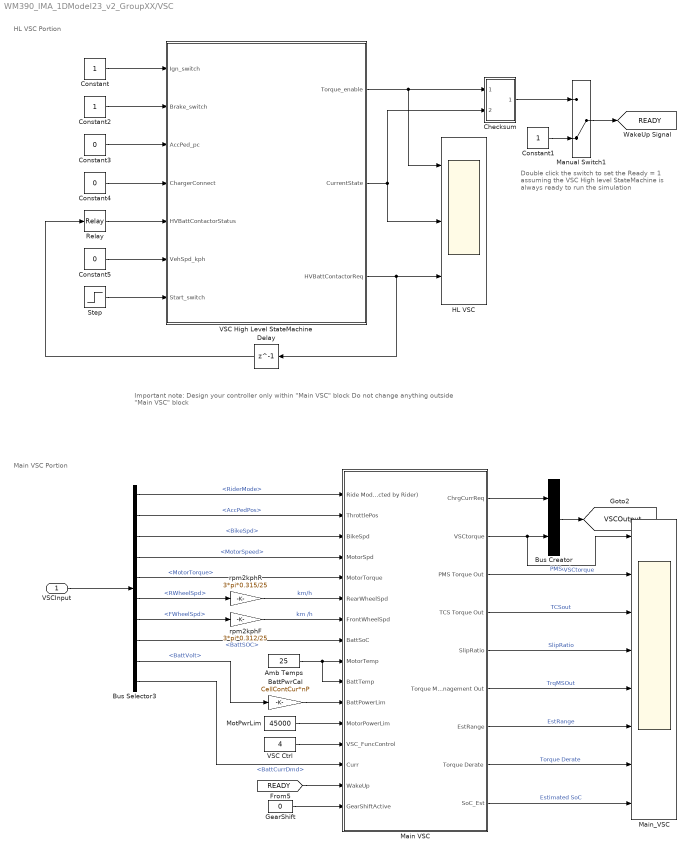
== system WM390_IMA_1DModel23_v2_GroupXX/VSC ==
  note: Double click the switch to set the Ready = 1
      | assuming the VSC High level StateMachine
      |  is always ready to run the simulation
  note: Main VSC Portion
  note: HL VSC Portion
  note: Important note:
      | Design your controller only within "Main VSC" block
      | Do not change anything outside "Main VSC" block
  VSCInput : Inport
  " VSC Ctrl" : Constant  Value=4
  Amb Temps : Constant  Value=25
  BattPwrCal : Gain  Gain=CellContCur*nP
  Bus Creator : BusCreator  Inputs=2  OutDataTypeStr=Bus: VSCBus
      settings: InheritFromInputs=off
  Bus Selector3 : BusSelector  OutputSignals=RiderCmd.RiderMode,AccPedPos,BikeSpd,MotorSpeed,MotorTorque,RWheelSpd,FWheelSpd,BatteryStates.BattSOC,BatteryStates.BattVolt,BattCurrDmd
  Checksum : Subsystem
  Constant : Constant
  Constant1 : Constant
  Constant2 : Constant
  Constant3 : Constant  Value=0
  Constant4 : Constant  Value=0
  Constant5 : Constant  Value=0
  Delay : Delay  DelayLength=1
  GearShift : Constant  Value=0
  HL VSC : Scope  NumInputPorts=3
  Main VSC : Subsystem
  Main_VSC : Scope  NumInputPorts=8
  Manual Switch1 : ManualSwitch  CurrentSetting=0
  MotPwrLim : Constant  Value=45000
  Relay : Relay  OnSwitchValue=1  OffSwitchValue=-1
  Step : Step  Time=5  Before=1  After=0  SampleTime=0
  VSC High Level StateMachine : Stateflow chart  TreatAsAtomicUnit=on
      settings: PortSchema="{\"entries\":[{\"content\":{\"sides\":[{\"content\":{\"connectorIds\":[\"In1\",\"In2\",\"In3\",\"In4\",\"In5\",\"In6\",\"In7\"]},\"type\":\"ConnectorPlacement.EquallySpacedRectSide\",\"uuid\":\"94b31f0f-cb33-4f9e-a39f-e19ad949fd84\"},{\"content\":{\"connectorIds\":[\"Out2\",\"Out3\",\"Out1\"],\"side\":\"RIGHT\"},\"type\":\"ConnectorPlacement.EquallySpacedRectSide\",\"uuid\":\"4fdac656-a6cd-488b-a850-0c9ed1c2a5fd\"},{\"content\":{\"connectorIds\":[],\"side\":\"TOP\"},\"type\":\"ConnectorPlacement.EquallySpacedRectSide\",\"uuid\":\"e7f633f9-4978-4bbb-80bf-32c0a2ef8aca\"}]},\"type\":\"ConnectorPlacement.EquallySpacedConnector\",\"uuid\":\"fa31f8e0-2942-414f-ad5d-d1693d30d12c\"}],\"packageUris\":[\"http://schema.mathworks.com/mf0/Connector/R2020b\"],\"version\":\"1.0\"}"
  rpm2kphF : Gain  Gain=3*pi*0.312/25
  rpm2kphR : Gain  Gain=3*pi*0.315/25
  tag scope: READY=global, VSCOutput=global
  wires:
  Main VSC/8(Torque Derate) -> Main_VSC/7  "Torque Derate"
  Main VSC/5(SlipRatio) -> Main_VSC/4  "SlipRatio"
  Main VSC/7(EstRange) -> Main_VSC/6  "EstRange"
  Main VSC/6("Torque Management Out ") -> Main_VSC/5  "TrqMSOut"
  Main VSC/3(PMS Torque Out) -> Main_VSC/2  "PMSout"
  Main VSC/4(TCS Torque Out) -> Main_VSC/3  "TCSout"
  Bus Creator/1 -> [VSCOutput]
  Manual Switch1/1 -> [READY]
  VSCInput/1 -> Bus Selector3/1
  Main VSC/2(VSCtorque) -> Main_VSC/1, Bus Creator/2  "VSCtorque"
  Checksum/1(Out1) -> Manual Switch1/1
  Constant1/1 -> Manual Switch1/2
  GearShift/1 -> Main VSC/16(GearShiftActive)
  Bus Selector3/4 -> Main VSC/4(MotorSpd)  "<MotorSpeed>"
  Bus Selector3/1 -> Main VSC/1(Ride Mode (Manually selected by Rider))  "<RiderMode>"
  Bus Selector3/2 -> Main VSC/2(ThrottlePos)  "<AccPedPos>"
  Bus Selector3/3 -> Main VSC/3(BikeSpd)  "<BikeSpd>"
  Bus Selector3/6 -> rpm2kphR/1  "<RWheelSpd>"
  Bus Selector3/7 -> rpm2kphF/1  "<FWheelSpd>"
  Amb Temps/1 -> Main VSC/10(BattTemp), Main VSC/9(MotorTemp)
  BattPwrCal/1 -> Main VSC/11(BattPowerLim)
  Bus Selector3/9 -> BattPwrCal/1  "<BattVolt>"
  " VSC Ctrl"/1 -> Main VSC/13(VSC_FuncControl)
  Bus Selector3/10 -> Main VSC/14(Curr)  "<BattCurrDmd>"
  rpm2kphR/1 -> Main VSC/6(RearWheelSpd)  "km/h"
  rpm2kphF/1 -> Main VSC/7(FrontWheelSpd)  "km /h"
  Main VSC/1(ChrgCurrReq) -> Bus Creator/1
  Bus Selector3/8 -> Main VSC/8(BattSoC)  "<BattSOC>"
  [READY] -> Main VSC/15(WakeUp)
  MotPwrLim/1 -> Main VSC/12(MotorPowerLim)
  Main VSC/9(SoC_Est) -> Main_VSC/8  "Estimated SoC"
  Bus Selector3/5 -> Main VSC/5(MotorTorque)  "<MotorTorque>"
  Delay/1 -> Relay/1
  Constant3/1 -> VSC High Level StateMachine/3(AccPed_pc)
  VSC High Level StateMachine/3(CurrentState) -> Checksum/2(CurrentState), HL VSC/2
  Constant5/1 -> VSC High Level StateMachine/6(VehSpd_kph)
  Constant2/1 -> VSC High Level StateMachine/2(Brake_switch)
  Step/1 -> VSC High Level StateMachine/7(Start_switch)
  VSC High Level StateMachine/2(Torque_enable) -> Checksum/1(Torque_enable), HL VSC/1
  Relay/1 -> VSC High Level StateMachine/5(HVBattContactorStatus)
  VSC High Level StateMachine/1(HVBattContactorReq) -> Delay/1, HL VSC/3
  Constant4/1 -> VSC High Level StateMachine/4(ChargerConnect)
  Constant/1 -> VSC High Level StateMachine/1(Ign_switch)

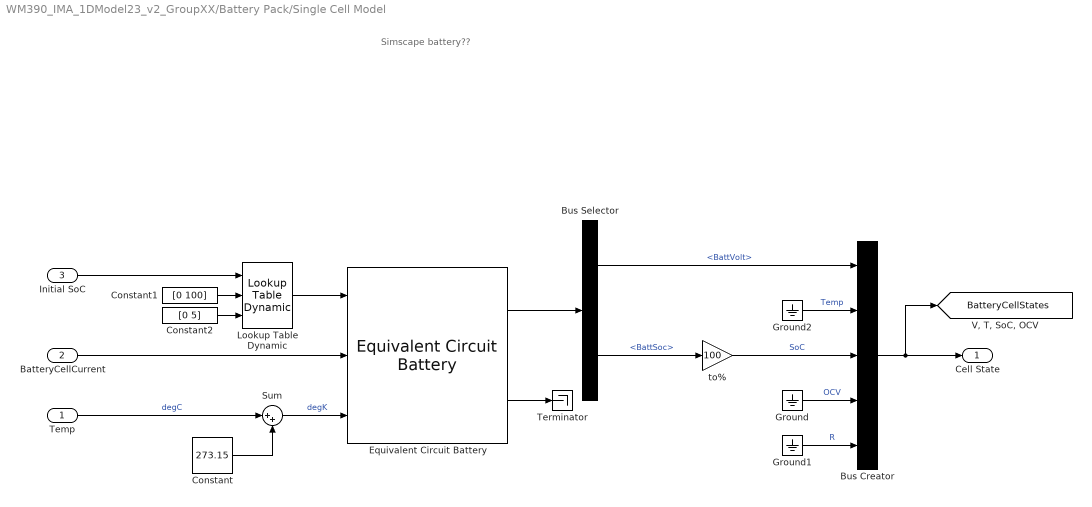
== system WM390_IMA_1DModel23_v2_GroupXX/Battery Pack/Single Cell Model ==
  note: Simscape battery??
  Temp : Inport
  BatteryCellCurrent : Inport  Port=2
  Initial SoC : Inport  Port=3
  Bus Creator : BusCreator  Inputs=5  OutDataTypeStr=Bus: CellStateBus
      settings: InheritFromInputs=off
  Bus Selector : BusSelector  OutputSignals=BattVolt,BattSoc
  Constant : Constant  Value=273.15
  Constant1 : Constant  Value=[0 100]
  Constant2 : Constant  Value=[0 5]
  Equivalent Circuit Battery : autolibrcnetworksystem/Equivalent Circuit Battery  CapacityCtrl=External Input  OutputVlt=Unfiltered  NumRC=1  Em=|  R0=|  SOC_BP=|  Temperature_BP=[293.15 313.15]  BattCap=[5 5]  BattCapInit=28  InitialCapVoltage=0  Tc=1/1000  Vinit=4.193  R1=|  C1=|  R2=|  C2=|  R3=|  C3=|  R4=|  C4=|  R5=|  C5=|  Vu=Inf  Vl=-Inf  RefBlkName='autolibrcnetworksystem/Equivalent Circuit Battery'
      Em=|
      | [3.5042 3.5136;
      | 3.5573 3.5646;
      | 3.6009 3.6153;
      | 3.6393 3.6565;
      | 3.6742 3.6889;
      | 3.7121 3.7214;
      | 3.7937 3.8078;
      | 3.8753 3.8945;
      | 3.97 3.9859;
      | 4.0764 4.0821;
      | 4.1924 4.193]
      R0=|
      | [0.011448 0.0090006;
      | 0.011038 0.0089655;
      | 0.011281 0.0091261;
      | 0.011236 0.0091099;
      | 0.010959 0.008957;
      | 0.010714 0.0087969;
      | 0.010698 0.0089126;
      | 0.010712 0.0090517;
      | 0.010917 0.0090444;
      | 0.011304 0.0088992;
      | 0.011603 0.0089015]
      SOC_BP=|
      | [0
      | 0.1
      | 0.2
      | 0.3
      | 0.4
      | 0.5
      | 0.6
      | 0.7
      | 0.8
      | 0.9
      | 1]
      R1=|
      | [0.010342 0.0012244;
      | 0.0067316 0.0011396;
      | 0.0051156 0.0012661;
      | 0.0043447 0.0012265;
      | 0.0038826 0.0011163;
      | 0.0034226 0.0009968;
      | 0.003346 0.0011458;
      | 0.0033222 0.001345;
      | 0.0033201 0.0013091;
      | 0.0032886 0.0010986;
      | 0.0028114 0.0010309]
      C1=|
      | [2287.7 11897;
      | 6122 24515;
      | 18460 42098;
      | 20975 44453;
      | 15254 33098;
      | 10440 24492;
      | 13903 32975;
      | 16694 40007;
      | 15784 35937;
      | 12165 26430;
      | 9118 24795]
      R2=|
      | [0.010342 0.0012244;
      | 0.0067316 0.0011396;
      | 0.0051156 0.0012661;
      | 0.0043447 0.0012265;
      | 0.0038826 0.0011163;
      | 0.0034226 0.0009968;
      | 0.003346 0.0011458;
      | 0.0033222 0.001345;
      | 0.0033201 0.0013091;
      | 0.0032886 0.0010986;
      | 0.0028114 0.0010309]
      C2=|
      | [2287.7 11897;
      | 6122 24515;
      | 18460 42098;
      | 20975 44453;
      | 15254 33098;
      | 10440 24492;
      | 13903 32975;
      | 16694 40007;
      | 15784 35937;
      | 12165 26430;
      | 9118 24795]
      R3=|
      | [0.010342 0.0012244;
      | 0.0067316 0.0011396;
      | 0.0051156 0.0012661;
      | 0.0043447 0.0012265;
      | 0.0038826 0.0011163;
      | 0.0034226 0.0009968;
      | 0.003346 0.0011458;
      | 0.0033222 0.001345;
      | 0.0033201 0.0013091;
      | 0.0032886 0.0010986;
      | 0.0028114 0.0010309]
      C3=|
      | [2287.7 11897;
      | 6122 24515;
      | 18460 42098;
      | 20975 44453;
      | 15254 33098;
      | 10440 24492;
      | 13903 32975;
      | 16694 40007;
      | 15784 35937;
      | 12165 26430;
      | 9118 24795]
      R4=|
      | [0.010342 0.0012244;
      | 0.0067316 0.0011396;
      | 0.0051156 0.0012661;
      | 0.0043447 0.0012265;
      | 0.0038826 0.0011163;
      | 0.0034226 0.0009968;
      | 0.003346 0.0011458;
      | 0.0033222 0.001345;
      | 0.0033201 0.0013091;
      | 0.0032886 0.0010986;
      | 0.0028114 0.0010309]
      C4=|
      | [2287.7 11897;
      | 6122 24515;
      | 18460 42098;
      | 20975 44453;
      | 15254 33098;
      | 10440 24492;
      | 13903 32975;
      | 16694 40007;
      | 15784 35937;
      | 12165 26430;
      | 9118 24795]
      R5=|
      | [0.010342 0.0012244;
      | 0.0067316 0.0011396;
      | 0.0051156 0.0012661;
      | 0.0043447 0.0012265;
      | 0.0038826 0.0011163;
      | 0.0034226 0.0009968;
      | 0.003346 0.0011458;
      | 0.0033222 0.001345;
      | 0.0033201 0.0013091;
      | 0.0032886 0.0010986;
      | 0.0028114 0.0010309]
      C5=|
      | [2287.7 11897;
      | 6122 24515;
      | 18460 42098;
      | 20975 44453;
      | 15254 33098;
      | 10440 24492;
      | 13903 32975;
      | 16694 40007;
      | 15784 35937;
      | 12165 26430;
      | 9118 24795]
      settings: SourceProductBaseCode=PW
  Ground : Ground
  Ground1 : Ground
  Ground2 : Ground
  Lookup Table Dynamic : simulink/Lookup Tables/Lookup Table Dynamic  LookUpMeth=Interpolation-Use End Values  OutDataType=fixdt('double')  OutScaling=[]  OutputDataTypeScalingMode=Specify via dialog  OutDataTypeStr=double  DoSatur=off
  Sum : Sum  Inputs=|++
  Terminator : Terminator
  to% : Gain  Gain=100
  Cell State : Outport  VectorParamsAs1DForOutWhenUnconnected=off
  tag scope: BatteryCellStates=global
  wires:
  Bus Creator/1 -> [BatteryCellStates], Cell State/1
  Ground2/1 -> Bus Creator/2  "Temp"
  Temp/1 -> Sum/1  "degC"
  Equivalent Circuit Battery/1 -> Bus Selector/1
  Bus Selector/1 -> Bus Creator/1  "<BattVolt>"
  Bus Selector/2 -> to%/1  "<BattSoc>"
  BatteryCellCurrent/1 -> Equivalent Circuit Battery/2
  Constant/1 -> Sum/2
  Sum/1 -> Equivalent Circuit Battery/3  "degK"
  Constant1/1 -> Lookup Table Dynamic/2
  Constant2/1 -> Lookup Table Dynamic/3
  Lookup Table Dynamic/1 -> Equivalent Circuit Battery/1
  Initial SoC/1 -> Lookup Table Dynamic/1
  to%/1 -> Bus Creator/3  "SoC"
  Ground/1 -> Bus Creator/4  "OCV"
  Ground1/1 -> Bus Creator/5  "R"
  Equivalent Circuit Battery/2 -> Terminator/1

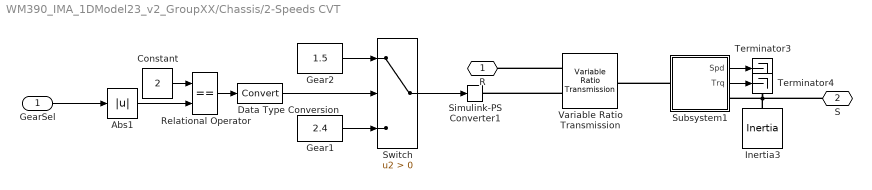
== system WM390_IMA_1DModel23_v2_GroupXX/Chassis/2-Speeds CVT ==
  GearSel : Inport
  Abs1 : Abs
  Constant : Constant  Value=2
  Data Type Conversion : DataTypeConversion
  Gear1 : Constant  Value=2.4
  Gear2 : Constant  Value=1.5
  Inertia3 : fl_lib/Mechanical/Rotational Elements/Inertia  inertia=0.001 kg*m^2  num_ports=foundation.enum.numPorts2.one  w_specify=off  w_priority=High  w=0 rad/s  w_nominal_specify=off  w_nominal_unit=rad/s  w_nominal_value=1  t_specify=off  t_priority=None  t=0 N*m  t_nominal_specify=off  t_nominal_unit=N*m  t_nominal_value=1
  Relational Operator : RelationalOperator  Operator===  OutDataTypeStr=boolean  RndMeth=Simplest
  Simulink-PS Converter1 : nesl_utility/Simulink-PS Converter  PhysicalDomain=network_engine_domain  SubClassName=ps_input  LeftPortType=input  RightPortType=output  PseudoPeriodic=off  Frequencies=[]  NoiseDistribution=none  NoiseParameters=[]  Unit=1  AffineConversion=off  FilteringAndDerivatives=provide  SimscapeFilterOrder=1  InputFilterTimeConstant=0.001  UdotUserProvided=0
      settings: SourceProductBaseCode=PW,SS
  Subsystem1 : Subsystem
      mask Display: disp('Rotational\nSensor 3')
  Switch : Switch  Criteria=u2 > Threshold
  Terminator3 : Terminator
  Terminator4 : Terminator
  Variable Ratio Transmission : sdl_lib/Couplings & Drives/Variable Ratio Transmission  rotation_direction=3-2*(2)  kp=3e5 N*m/rad  kv=0.0005 N*m/(rad/s)  initial_torque=0 N*m  losses_model=(1)-1  efficiency=RatioEfficiency  w_thr=0.0001 rad/s  mu_visc=[0, 0] N*m/(rad/s)  R_specify=off  R_priority=None  R=1  R_nominal_specify=off  R_nominal_unit=1  R_nominal_value=1
      settings: SourceProductBaseCode=LD  InternalSimscapePortConfiguration="{\"Bottom\":[],\"Left\":[{\"id\":\"ratio\",\"label\":\"r\",\"type\":\"input\"},{\"id\":\"B\",\"label\":\"B\",\"type\":\"foundation.mechanical.rotational.rotational\"}],\"Right\":[{\"id\":\"F\",\"label\":\"F\",\"type\":\"foundation.mechanical.rotational.rotational\"}],\"Top\":[]}"
  R : PMIOPort  Side=Left
  S : PMIOPort  Port=2  Side=Right
  wires:
  Gear1/1 -> Switch/3
  Subsystem1/2(Trq) -> Terminator4/1
  Gear2/1 -> Switch/1
  Switch/1 -> Simulink-PS Converter1/1
  Subsystem1/1(Spd) -> Terminator3/1
  Relational Operator/1 -> Data Type Conversion/1
  Abs1/1 -> Relational Operator/2
  Constant/1 -> Relational Operator/1
  Data Type Conversion/1 -> Switch/2
  GearSel/1 -> Abs1/1
  connections:
  Variable Ratio Transmission/LConn2 -- R/RConn1
  Subsystem1/LConn1 -- Variable Ratio Transmission/RConn1
  Inertia3/LConn1 -- S/RConn1 -- Subsystem1/RConn1
  Variable Ratio Transmission/LConn1 -- Simulink-PS Converter1/RConn1

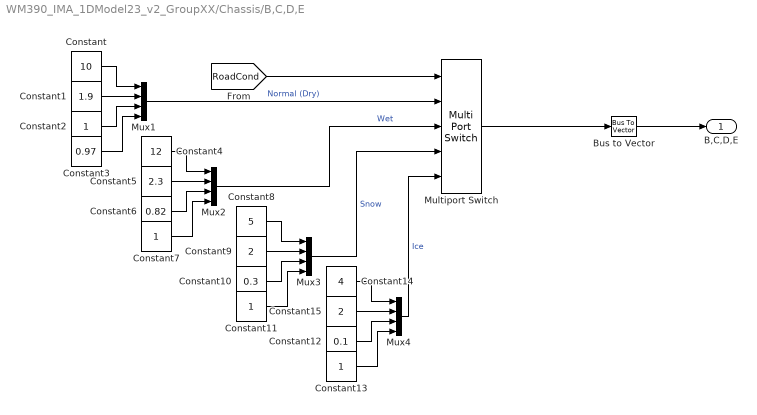
== system WM390_IMA_1DModel23_v2_GroupXX/Chassis/B,C,D,E ==
  Bus to Vector : BusToVector
  Constant : Constant  Value=10
  Constant1 : Constant  Value=1.9
  Constant10 : Constant  Value=0.3
  Constant{2,7,11,13} (4 alike) : Constant
  Constant12 : Constant  Value=0.1
  Constant14 : Constant  Value=4
  Constant15 : Constant  Value=2
  Constant3 : Constant  Value=0.97
  Constant4 : Constant  Value=12
  Constant5 : Constant  Value=2.3
  Constant6 : Constant  Value=0.82
  Constant8 : Constant  Value=5
  Constant9 : Constant  Value=2
  Multiport Switch : MultiPortSwitch  Inputs=4
  Mux{1..4} (4 alike) : Mux
  B,C,D,E : Outport
  wires:
  Bus to Vector/1 -> B,C,D,E/1
  Constant1/1 -> Mux1/2
  Constant/1 -> Mux1/1
  Constant3/1 -> Mux1/4
  Constant2/1 -> Mux1/3
  Mux1/1 -> Multiport Switch/2  "Normal (Dry)"
  Multiport Switch/1 -> Bus to Vector/1
  [RoadCond] -> Multiport Switch/1
  Mux2/1 -> Multiport Switch/3  "Wet"
  Constant6/1 -> Mux2/3
  Constant7/1 -> Mux2/4
  Constant4/1 -> Mux2/1
  Constant5/1 -> Mux2/2
  Constant9/1 -> Mux3/2
  Constant8/1 -> Mux3/1
  Constant11/1 -> Mux3/4
  Constant10/1 -> Mux3/3
  Mux3/1 -> Multiport Switch/4  "Snow"
  Mux4/1 -> Multiport Switch/5  "Ice"
  Constant12/1 -> Mux4/3
  Constant13/1 -> Mux4/4
  Constant14/1 -> Mux4/1
  Constant15/1 -> Mux4/2

== system WM390_IMA_1DModel23_v2_GroupXX/Chassis/Subsystem1 ==
  Ideal Rotational Motion Sensor : fl_lib/Mechanical/Mechanical Sensors/Ideal Rotational Motion Sensor  wrap_angle=simscape.enum.onoff.off  offset=0 rad
  Ideal Torque Sensor : fl_lib/Mechanical/Mechanical Sensors/Ideal Torque Sensor
  Mechanical Rotational Reference1 : fl_lib/Mechanical/Rotational Elements/Mechanical Rotational Reference
  PS-Simulink Converter : nesl_utility/PS-Simulink Converter  PhysicalDomain=network_engine_domain  SubClassName=ps_output  LeftPortType=input  RightPortType=output  PseudoPeriodic=off  Frequencies=[]  Unit=N*m  AffineConversion=off
      settings: SourceProductBaseCode=PW,SS
  PS-Simulink Converter1 : nesl_utility/PS-Simulink Converter  PhysicalDomain=network_engine_domain  SubClassName=ps_output  LeftPortType=input  RightPortType=output  PseudoPeriodic=off  Frequencies=[]  Unit=rpm  AffineConversion=off
      settings: SourceProductBaseCode=PW,SS
  PS-Simulink Converter2 : nesl_utility/PS-Simulink Converter  PhysicalDomain=network_engine_domain  SubClassName=ps_output  LeftPortType=input  RightPortType=output  PseudoPeriodic=off  Frequencies=[]  Unit=1  AffineConversion=off
      settings: SourceProductBaseCode=PW,SS
  Terminator2 : Terminator
  Terminator3 : Terminator
  Conn1 : PMIOPort  Side=Right
  Conn2 : PMIOPort  Port=2  Side=Left
  RWSpd : Outport
  wires:
  PS-Simulink Converter2/1 -> Terminator2/1  "WheelRrAcc"
  PS-Simulink Converter/1 -> Terminator3/1  "WheelRrTq"
  PS-Simulink Converter1/1 -> RWSpd/1  "RWSpd [rpm]"
  connections:
  Ideal Rotational Motion Sensor/RConn3 -- PS-Simulink Converter2/LConn1
  PS-Simulink Converter/LConn1 -- Ideal Torque Sensor/RConn2
  PS-Simulink Converter1/LConn1 -- Ideal Rotational Motion Sensor/RConn2
  Mechanical Rotational Reference1/LConn1 -- Ideal Rotational Motion Sensor/RConn1
  Ideal Rotational Motion Sensor/LConn1 -- Ideal Torque Sensor/RConn1 -- Conn1/RConn1
  Ideal Torque Sensor/LConn1 -- Conn2/RConn1
